simulink model "TransmissionLine_AC_System"  (R2024b)
settings: Solver=ode1be  StartTime=0.0  StopTime=tfinal  FixedStep=dt_sim  RelTol=1e-6
values from neighbouring files (symbols this model uses):
  dt_sim = 1e-6    (= 1e-06)    [Ex_AC_System.m]
  Line_num = 10    [Ex_AC_System.m]
libraries: spsPiSectionLineLib x11, spsGroundLib x2, spsCurrentMeasurementLib x1, spsSeriesRLCLoadLib x1, spsACVoltageSourceLib x1, spsSeriesRLCBranchLib x1, spspowerguiLib x1, spsVoltageMeasurementLib x1
settings Model: Creator=The MathWorks, Inc.  LastModifiedBy=wei13
settings SolverCC: AlgebraicLoopSolver=TrustRegion
settings DataIOCC: SaveFormat=Array  ReturnWorkspaceOutputs=off  SignalLoggingName=sigsOut
settings OptimizationCC: BlockReduction=off  BooleanDataType=off  ExpressionDepthLimit=2147483647  InitFltsAndDblsToZero=on  EfficientMapNaN2IntZero=off  LifeSpan=inf
settings DebuggingCC: AlgebraicLoopMsg=none  SaveWithParameterizedLinksMsg=none  UnderspecifiedInitializationDetection=Classic  MergeDetectMultiDrivingBlocksExec=none  CheckExecutionContextPreStartOutputMsg=on  SignalResolutionControl=TryResolveAllWithWarning  MultiTaskDSMMsg=warning  MultiTaskCondExecSysMsg=none  SigSpecEnsureSampleTimeMsg=none  FcnCallInpInsideContextMsg=warning  StateNameClashWarn=warning  SFUnexpectedBacktrackingDiag=warning  SFNoUnconditionalDefaultTransitionDiag=warning  SFExecutionAtInitializationDiag=none  ArithmeticOperatorsInVariantConditions=warning
settings HardwareCC: ProdBitPerPointer=32  ProdBitPerSizeT=32  ProdBitPerPtrDiffT=32  ProdLargestAtomicFloat=None  ProdIntDivRoundTo=Undefined  ProdEndianess=Unspecified  ProdWordSize=32  ProdHWDeviceType=32-bit Generic  TargetUnknown=on
settings ModelReferenceCC: EnableRefExpFcnMdlSchedulingChecks=on  PropagateSignalLabelsOutOfModel=off
settings SFSimCC: SimUseLocalCustomCode=off  CustomCodeUndefinedFunction=UseInterfaceOnly
settings RTWCC: RTWUseLocalCustomCode=off  GPUComputeCapability=3.5  DLArmComputeVersion=19.05
settings CodeAppCC: StateflowObjectComments=on
settings GRTTargetCC: TargetFcnLib=ansi_tfl_tmw.mat  TargetLangStandard=C89/C90 (ANSI)  CombineOutputUpdateFcns=off  GRTInterface=on
settings ConfigComp: CovMetricSettings=dw  CovSaveCumulativeToWorkspaceVar=on  CovSaveSingleToWorkspaceVar=on  CovExternalEMLEnable=off  CovSFcnEnable=off
settings SimscapeCC: SimscapeNormalizeSystem=off

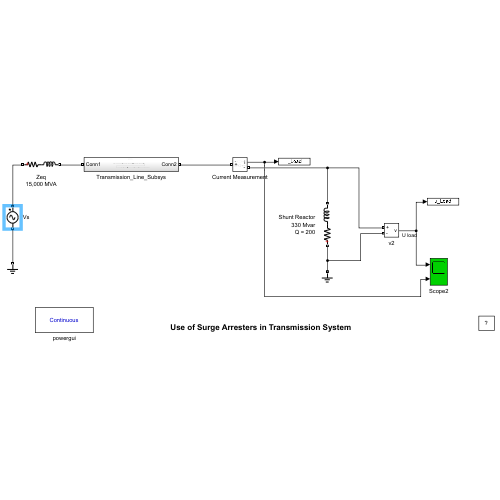
[thumbnail: Simulink's stored preview of the top-level diagram]
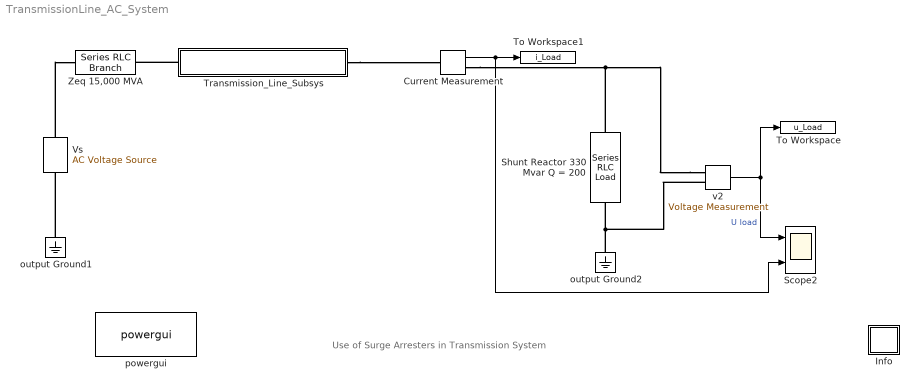
== system TransmissionLine_AC_System ==
  note: Use of Surge Arresters in Transmission System
  Current Measurement : spsCurrentMeasurementLib/Current Measurement  PhasorSimulation=off  OutputType=Complex  PSBequivalent=0
  Info : Subsystem
      settings: OpenFcn="showExample(\"simscapeelectricalsps/SurgeArrestersExample\")"
      mask Display: disp('?')
  Scope2 : Scope  NumInputPorts=2
  Shunt Reactor 330 Mvar Q = 200 : spsSeriesRLCLoadLib/Series RLC Load  LConnTagsString=a  RConnTagsString=__new0  NominalVoltage=735e3/sqrt(3)  NominalFrequency=60  ActivePower=330e6/3/200  InductivePower=330e6/3  CapacitivePower=0  Setx0=off  InitialVoltage=0  SetiL0=off  InitialCurrent=0  Measurements=None  LoadType=constant Z
  To Workspace : ToWorkspace  VariableName=u_Load  SampleTime=-1
      settings: Save2DSignal=2-D array (concatenate along first dimension)
  To Workspace1 : ToWorkspace  VariableName=i_Load  SampleTime=-1
      settings: Save2DSignal=2-D array (concatenate along first dimension)
  Transmission_Line_Subsys : Subsystem
  Vs : spsACVoltageSourceLib/AC Voltage Source  Description=source block  Amplitude=735e3/sqrt(3)*sqrt(2)  Phase=0  Frequency=60  SampleTime=0  Measurements=None  BusType=swing  Pref=10e3  Qref=0  Qmin=-inf  Qmax=+inf
      settings: AttributesFormatString=\n
  Zeq 15,000 MVA : spsSeriesRLCBranchLib/Series RLC Branch  LConnTagsString=__new0  RConnTagsString=__new0  BranchType=RL  Resistance=3.6  Inductance=95.5e-3  SetiL0=off  InitialCurrent=0  Capacitance=[]  Setx0=off  InitialVoltage=0  Measurements=None
  output Ground1 : spsGroundLib/Ground  LConnTagsString=a
  output Ground2 : spsGroundLib/Ground  LConnTagsString=a
  powergui : spspowerguiLib/powergui  Priority=2  SimulationMode=Continuous  SampleTime=dt_sim  frequency=60  Iterations=50  frequencyindice=60  Pbase=100e6  ErrMax=1e-4  UnitsV=kV  UnitsW=MW  buscounter=0  FunctionMessages=off  echomessages=off  EnableUseOfTLC=off  CurrentSourceSwitches=off  DisableSnubberDevices=on  DisableRonSwitches=off  DisableVfSwitches=off  DisplayEquations=off  AutomaticDiscreteSolvers=off  SolverType=Tustin  Interpol=off  ExternalGateDelay=off  methode=off  Ts=0  x0status=blocks  SPID=on  SwTol=0  HookPort=off  NonlinearTolerance=1e-4  nMaxIteration=100  ContinueOnMaxIteration=off  RestoreLinks=warning  ResistiveCurrentMeasurement=off  Frange=logspace(0,3,50)  Ylog=off  Xlog=off  ShowGrid=off  save=off  variable=ZData  structure=0  ZoomFFT=on  StartTime=0.0  cycles=1  DisplayStyle=off  fundamental=60  FreqAxis=off  MaxFrequency=1000  frequencyindicesteady=1  RmsSteady=1  display=off
  v2 : spsVoltageMeasurementLib/Voltage Measurement  Tag=PoWeRsYsTeMmEaSuReMeNt  PhasorSimulation=off  OutputType=Magnitude  PSBequivalent=0
  wires:
  v2/1 -> To Workspace/1, Scope2/1  "U load"
  Current Measurement/1 -> Scope2/2, To Workspace1/1
  connections:
  output Ground1/LConn1 -- Vs/LConn1
  Vs/RConn1 -- Zeq 15,000 MVA/LConn1
  output Ground2/LConn1 -- Shunt Reactor 330 Mvar Q = 200/LConn1 -- v2/LConn2
  v2/LConn1 -- Current Measurement/RConn1 -- Shunt Reactor 330 Mvar Q = 200/RConn1
  Transmission_Line_Subsys/LConn1 -- Zeq 15,000 MVA/RConn1
  Transmission_Line_Subsys/RConn1 -- Current Measurement/LConn1

== system TransmissionLine_AC_System/Info ==

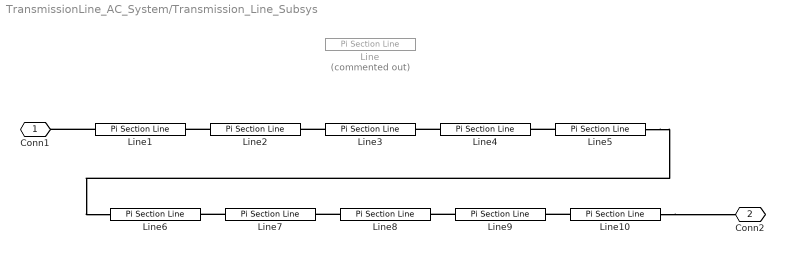
== system TransmissionLine_AC_System/Transmission_Line_Subsys ==
  Line : spsPiSectionLineLib/Pi Section Line  Commented=on  LConnTagsString=__new0  RConnTagsString=__new0  Phases=1  PiSections=2*Line_num  Length=200  Frequency=60  Resistance=0.011  Inductance=0.8674e-3  Capacitance=13.41e-9  SpecifyConductance=off  Conductance=0  Measurements=None  Measurements2=None
  Line{1..10} (10 alike) : spsPiSectionLineLib/Pi Section Line  LConnTagsString=__new0  RConnTagsString=__new0  Phases=1  PiSections=2  Length=200/Line_num  Frequency=60  Resistance=0.011  Inductance=0.8674e-3  Capacitance=13.41e-9  SpecifyConductance=off  Conductance=0  Measurements=None  Measurements2=None
  Conn1 : PMIOPort  Side=Left
  Conn2 : PMIOPort  Port=2  Side=Right
  connections:
  Line5/LConn1 -- Line4/RConn1
  Line2/LConn1 -- Line1/RConn1
  Line3/LConn1 -- Line2/RConn1
  Line4/LConn1 -- Line3/RConn1
  Line7/LConn1 -- Line6/RConn1
  Line8/LConn1 -- Line7/RConn1
  Line9/LConn1 -- Line8/RConn1
  Line10/LConn1 -- Line9/RConn1
  Line5/RConn1 -- Line6/LConn1
  Line10/RConn1 -- Conn2/RConn1
  Line1/LConn1 -- Conn1/RConn1
